simulink model "carriers_ASK_BPSK"  (R2022b)
settings: Solver=VariableStepDiscrete  StartTime=0.0  StopTime=tsim  RelTol=1e-3
values from neighbouring files (symbols this model uses):
  Ac = 1    [init_vars.m]
  fc = 10e3    (= 10000)    [init_vars.m]
  fs = spb * rb    (= 100000)    [init_vars.m]
  rb = 1e3    (= 1000)    [init_vars.m]
  rng_seed = 5    [init_vars.m]
  spb = 100    [init_vars.m]
libraries: dspsigops x2, commrandsrc3 x1, commutil2 x1
settings Model: Creator=pedro  LastModifiedBy=joaogaspar
settings SolverCC: AlgebraicLoopSolver=TrustRegion
settings DebuggingCC: UnconnectedInputMsg=warning  UnconnectedOutputMsg=warning  UnconnectedLineMsg=warning  SFMachineParentedDataDiag=warning
settings ModelReferenceCC: EnableRefExpFcnMdlSchedulingChecks=on

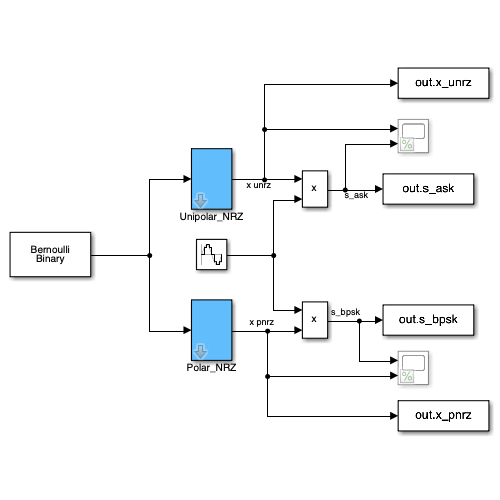
[thumbnail: Simulink's stored preview of the top-level diagram]
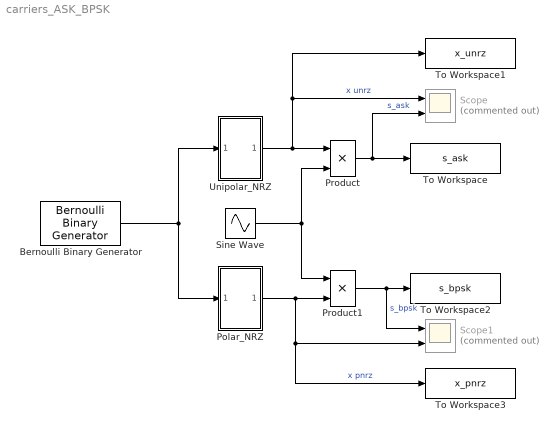
== system carriers_ASK_BPSK ==
  Bernoulli Binary Generator : commrandsrc3/Bernoulli Binary Generator  ProbabilityOfZero=0.5  SeedSource=Parameter  Seed=rng_seed  SampleTime=1/rb  SamplesPerFrame=1  OutputDataType=double  SimulateUsing=Interpreted execution
  Polar_NRZ : Subsystem  mask(Polar_nrz){Rb=rb, Spb=spb}
      mask prompts: Rb "Binary Data Rate"; Spb "Samples per bit"
  Product : Product
  Product1 : Product
  Scope : Scope  Commented=on  NumInputPorts=2
  Scope1 : Scope  Commented=on  NumInputPorts=2
  Sine Wave : Sin  Amplitude=Ac  Frequency=2*pi*fc  SampleTime=1/fs
  To Workspace : ToWorkspace  VariableName=s_ask  SaveFormat=Timeseries  SampleTime=-1
  To Workspace1 : ToWorkspace  VariableName=x_unrz  SaveFormat=Timeseries  SampleTime=-1
  To Workspace2 : ToWorkspace  VariableName=s_bpsk  SaveFormat=Timeseries  SampleTime=-1
  To Workspace3 : ToWorkspace  VariableName=x_pnrz  SaveFormat=Timeseries  SampleTime=-1
  Unipolar_NRZ : Subsystem  mask(unipolar_nrz){Rb=rb, Spb=spb}
      mask prompts: Rb "Binary Data Rate"; Spb "Samples per bit"
  wires:
  Sine Wave/1 -> Product/2, Product1/1
  Unipolar_NRZ/1(Out1) -> To Workspace1/1, Scope/1, Product/1  "x unrz"
  Product/1 -> Scope/2, To Workspace/1  "s_ask"
  Bernoulli Binary Generator/1 -> Unipolar_NRZ/1(In1), Polar_NRZ/1(In1)
  Polar_NRZ/1(Out1) -> Product1/2, Scope1/2, To Workspace3/1  "x pnrz"
  Product1/1 -> Scope1/1, To Workspace2/1  "s_bpsk"

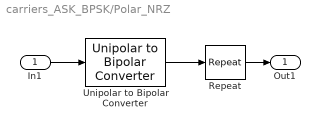
== system carriers_ASK_BPSK/Polar_NRZ ==
  In1 : Inport
  Repeat : dspsigops/Repeat  N=Spb  InputProcessing=Columns as channels (frame based)  RateOptions=Allow multirate processing  ic=0  mode=Unused parameter value
  Unipolar to Bipolar Converter : commutil2/Unipolar to Bipolar Converter  M=2  polarity=Positive  dataType=Same as input
  Out1 : Outport
  wires:
  Unipolar to Bipolar Converter/1 -> Repeat/1
  In1/1 -> Unipolar to Bipolar Converter/1
  Repeat/1 -> Out1/1

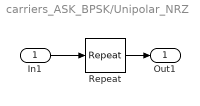
== system carriers_ASK_BPSK/Unipolar_NRZ ==
  In1 : Inport
  Repeat : dspsigops/Repeat  N=Spb  InputProcessing=Columns as channels (frame based)  RateOptions=Allow multirate processing  ic=0  mode=Unused parameter value
  Out1 : Outport
  wires:
  In1/1 -> Repeat/1
  Repeat/1 -> Out1/1
